simulink model "Anfis_sist_no_lineal"  (R2016a)
settings: Solver=VariableStepAuto  StartTime=0.0  StopTime=200  RelTol=1e-3
values from neighbouring files (symbols this model uses):
  b = [1;1]    [ejemplodiscretro.m]
undefined symbols (not defined in the file or in its folder): k
settings Model: Creator=Daniel  LastModifiedBy=Daniel

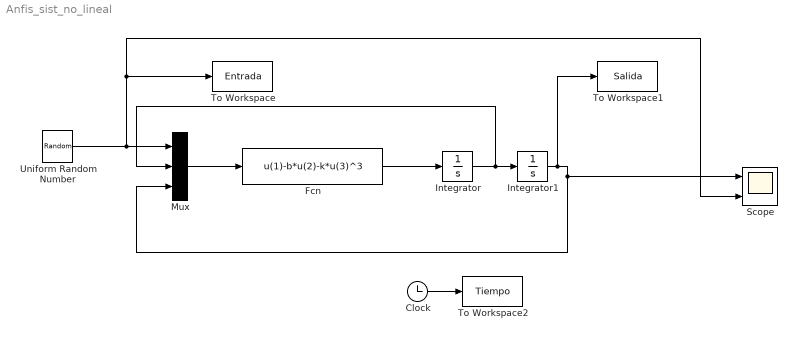
== system Anfis_sist_no_lineal ==
  Clock : Clock
  Fcn : Fcn  Expr=u(1)-b*u(2)-k*u(3)^3
  Integrator : Integrator
  Integrator1 : Integrator
  Mux : Mux  Inputs=3
  Scope : Scope  NumInputPorts=2
  To Workspace : ToWorkspace  VariableName=Entrada  SampleTime=0.1
  To Workspace1 : ToWorkspace  VariableName=Salida  SampleTime=0.1
  To Workspace2 : ToWorkspace  VariableName=Tiempo  SampleTime=0.1
  Uniform Random Number : UniformRandomNumber  Minimum=0  Maximum=5  SampleTime=10
  wires:
  Mux/1 -> Fcn/1
  Fcn/1 -> Integrator/1
  Integrator/1 -> Mux/2, Integrator1/1
  Integrator1/1 -> To Workspace1/1, Scope/1, Mux/3
  Uniform Random Number/1 -> Scope/2, To Workspace/1, Mux/1
  Clock/1 -> To Workspace2/1
